simulink model "mltvlib_tvss"  (R2018b)
settings: Solver=VariableStepAuto  StartTime=0.0  StopTime=10.0  RelTol=1e-3
undefined symbols (not defined in the file or in its folder): Asys, Atvsys, Bsys, Btvsys, Csys, Ctvsys, Dsys, Dtvsys, x0sys
libraries: ltvlib x1
settings Model: Creator=jyotbuch  LastModifiedBy=jyotbuch

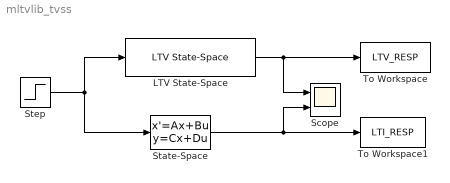
== system mltvlib_tvss ==
  LTV State-Space : ltvlib/LTV State-Space  A=Atvsys  B=Btvsys  C=Ctvsys  D=Dtvsys  x0=x0tvsys
      settings: SourceProductName=Linear Time-Varying Systems Toolbox
  Scope : Scope  NumInputPorts=2
  State-Space : StateSpace  A=Asys  B=Bsys  C=Csys  D=Dsys  InitialCondition=x0sys
  Step : Step  SampleTime=0
  To Workspace : ToWorkspace  VariableName=LTV_RESP  SampleTime=-1
  To Workspace1 : ToWorkspace  VariableName=LTI_RESP  SampleTime=-1
  wires:
  Step/1 -> LTV State-Space/1, State-Space/1
  State-Space/1 -> To Workspace1/1, Scope/2
  LTV State-Space/1 -> To Workspace/1, Scope/1
